simulink model "sldemo_tonegen_fixpt"  (Simulink 6.0)
settings: Solver=FixedStepDiscrete  SolverMode=SingleTasking  StartTime=0  StopTime=30  FixedStep=1/256  RelTol=1e-3
StopFcn:
  | subplot(2,1,1), plot(tonegenOut.time, tonegenOut.signals(1).values); grid
  | subplot(2,1,2), plot(tonegenOut.time, tonegenOut.signals(2).values); grid
libraries: simulink x4
settings Model: Creator=The MathWorks Inc.  LastModifiedBy=batserve  ExtModeAutoUpdateStatusClock=off
settings DataIOCC: LimitDataPoints=off  SaveFormat=StructureWithTime  SaveTime=off  OutputSaveName=tonegenOut  SignalLoggingName=sigsOut
settings DebuggingCC: CheckExecutionContextPreStartOutputMsg=on  CheckExecutionContextRuntimeOutputMsg=on  SolverPrmCheckMsg=none
settings HardwareCC: TargetUnknown=on

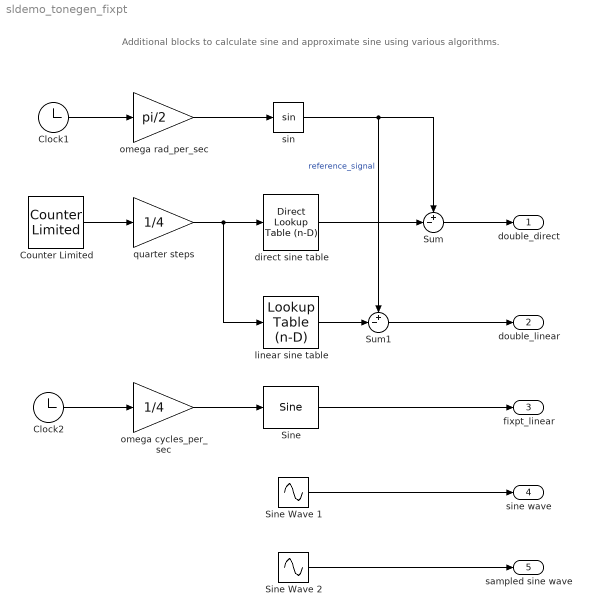
== system sldemo_tonegen_fixpt ==
  note: Additional blocks to calculate sine and
      | approximate sine using various algorithms.
  Clock1 : Clock
      settings: Decimation=10
  Clock2 : Clock
      settings: Decimation=10
  Counter Limited : simulink/Sources/Counter Limited  uplimit=1023  tsamp=-1
  Sine : simulink/Lookup Tables/Sine  NumDataPoints=(2^5)+1
  Sine Wave 1 : Sin  SampleTime=0
  Sine Wave 2 : Sin  SineType=Sample based  Frequency=pi/2  SampleTime=1/256
  Sum : Sum  Inputs=+-|
  Sum1 : Sum  Inputs=+-|
  direct sine table : simulink/Lookup Tables/Direct Lookup Table (n-D)  maskTabDims=1  explicitNumDims=1  outDims=Element  tabIsInput=off  mxTable=sin( 2*pi * (0:255)/256)'  clipFlag=Warning
  linear sine table : simulink/Lookup Tables/Lookup Table (n-D)  numDimsPopupSelect=1  bp1=[0:256]  bp2=[10,22,31]  bp3=[1:3]  bp4=[1:3]  bpcell={ [1:3], [1:3] }  explicitNumDims=2  searchMode=Linear Search  cacheBpFlag=on  vectorInputFlag=off  tableData=sin( 2*pi * (0:256)/256 )'  interpMethod=Linear  extrapMethod=None - Clip  rangeErrorMode=Warning
  omega cycles_per_sec : Gain  Gain=1/4
  omega rad_per_sec : Gain  Gain=pi/2
  quarter steps : Gain  Gain=1/4  OutDataTypeMode=Specify via dialog  OutDataType=float('double')
  sin : Trigonometry
  double_direct : Outport
  double_linear : Outport  Port=2
  fixpt_linear : Outport  Port=3
  sine wave : Outport  Port=4
  sampled sine wave : Outport  Port=5
  wires:
  Clock1/1 -> omega rad_per_sec/1
  omega rad_per_sec/1 -> sin/1
  Counter Limited/1 -> quarter steps/1
  quarter steps/1 -> direct sine table/1, linear sine table/1
  sin/1 -> Sum/1, Sum1/1  "reference_signal"
  direct sine table/1 -> Sum/2
  linear sine table/1 -> Sum1/2
  Sum/1 -> double_direct/1
  Sum1/1 -> double_linear/1
  Sine/1 -> fixpt_linear/1
  Clock2/1 -> omega cycles_per_sec/1
  omega cycles_per_sec/1 -> Sine/1
  Sine Wave 1/1 -> sine wave/1
  Sine Wave 2/1 -> sampled sine wave/1
